simulink model "OpticalFlow"  (Simulink 10.0)
settings: Solver=ode45  StartTime=0.0  StopTime=inf  RelTol=1e-3  EnableMultiTasking=on
undefined symbols (not defined in the file): Horn, Schunck, strel
libraries: vipsnks x4, dspstat3 x2, vipstatistics x1, vipmorphops x1, viptextngfix x1, dspsrcs4 x1, vipanalysis x1
settings Model: Creator=ahwang  LastModifiedBy=bhisma
settings SolverCC: ZeroCrossAlgorithm=Non-adaptive
settings DataIOCC: LimitDataPoints=on  SignalLoggingSaveFormat=ModelDataLogs
settings OptimizationCC: ExpressionDepthLimit=2147483647  InitFltsAndDblsToZero=on
settings DebuggingCC: SolverPrmCheckMsg=warning  FcnCallInpInsideContextMsg=warning  StateNameClashWarn=warning
settings SFSimCC: SimUseLocalCustomCode=on  SimParseCustomCode=off  CustomCodeUndefinedFunction=FilterOut
settings RTWCC: RTWUseLocalCustomCode=on

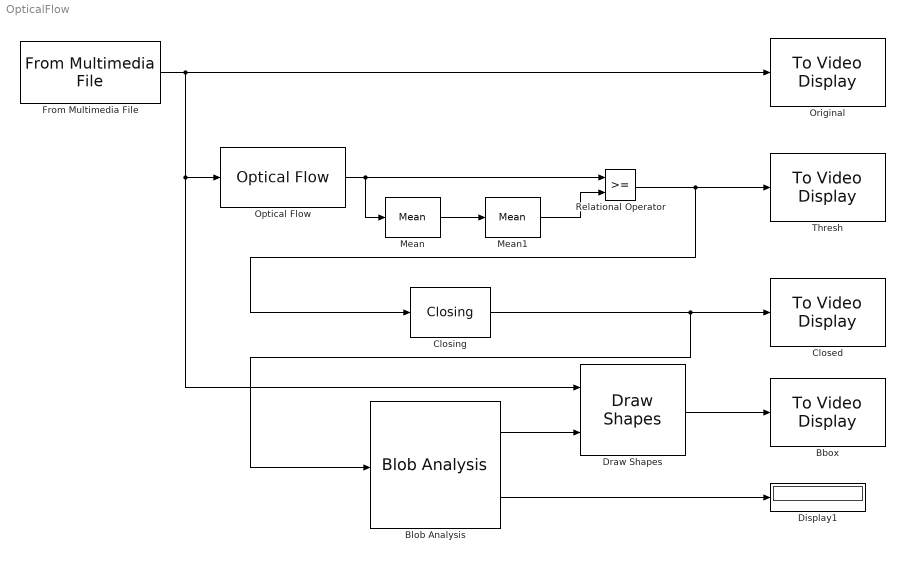
== system OpticalFlow ==
  Bbox : vipsnks/To Video Display  inputType=Obsolete  imagePorts=One multidimensional signal  OutputDevice=On-screen video monitor  fullScreen=off  videoWindowX=289  videoWindowY=479  saveWindowSize=off  videoWindowWidth=44  videoWindowHeight=41  dataOrg=Column-major
      settings: SourceProductName=Computer Vision Toolbox  SourceProductBaseCode=VP
  Blob Analysis : vipstatistics/Blob Analysis  area=off  centroid=off  bBox=on  majorAxis=off  minorAxis=off  angle=off  eccentricity=off  equivDiameterSq=off  extent=off  perimeter=off  maxBlobs=50  warnIfNumBlobsExceeded=on  isCount=on  useMinArea=on  minArea=200  useMaxArea=off  maxArea=intmax('uint32')  excludeBorderBlob=off  outDT=double  isOutVarDim=off  isFill=on  fillValues=-1  conn=8  isLabel=off  outputMode=Binary point scaling  outputWordLength=32  outputFracLength=16  firstCoeffMode=Binary point scaling  firstCoeffWordLength=16  firstCoeffFracLength=14  secondCoeffMode=Binary point scaling  secondCoeffWordLength=32  secondCoeffFracLength=16  accumMode=Binary point scaling  accumWordLength=32  accumFracLength=0  prodOutputMode=Binary point scaling  prodOutputWordLength=32  prodOutputFracLength=16  roundingMode=Floor  overflowMode=off
      settings: SourceProductName=Computer Vision Toolbox  SourceProductBaseCode=VP
  Closed : vipsnks/To Video Display  inputType=Obsolete  imagePorts=One multidimensional signal  OutputDevice=On-screen video monitor  fullScreen=off  videoWindowX=292  videoWindowY=332  saveWindowSize=off  videoWindowWidth=44  videoWindowHeight=41  dataOrg=Column-major
      settings: SourceProductName=Computer Vision Toolbox  SourceProductBaseCode=VP
  Closing : vipmorphops/Closing  nhoodsrc=Specify via dialog  strel=strel('disk',5)
      settings: SourceProductName=Computer Vision Toolbox  SourceProductBaseCode=VP
  Display1 : Display
  Draw Shapes : viptextngfix/Draw Shapes  shape=Rectangles  fill=off  display=Black  intensity=200  color=[200 255 100]  opacity=0.6  viewport=Entire image  antialiasing=off  inType=Obsolete  imagePorts=One multidimensional signal
      settings: SourceProductName=Computer Vision Toolbox  SourceProductBaseCode=VP
  From Multimedia File : dspsrcs4/From Multimedia File  inputFilename=viptraffic.avi  loop=on  numPlays=inf  outputStreams=Video only  videoDataType=double  audioDataType=int16  inheritSampleTime=on  userDefinedSampleTime=1/30  noAudioOutput=off  isIntensityVideo=on  colorVideoFormat=One multidimensional signal  outputEOF=off  dataOrg=Column-major
      settings: SourceProductName=DSP System Toolbox  SourceProductBaseCode=DS
  Mean : dspstat3/Mean  run=off  reset_popup=None  directionMode=Entire input  dimension=1  treatSBRowAsCol=on  roiEnable=off  roiType=Rectangles  roiPortion=Entire ROI  roiOutput=Individual statistics for each ROI  roiFlag=off  roundingMode=Floor  overflowMode=off
  Mean1 : dspstat3/Mean  run=on  reset_popup=None  directionMode=Entire input  dimension=1  treatSBRowAsCol=on  roiEnable=off  roiType=Rectangles  roiPortion=Entire ROI  roiOutput=Individual statistics for each ROI  roiFlag=off  roundingMode=Floor  overflowMode=off
  Optical Flow : vipanalysis/Optical Flow  SystemSampleTime=-1  method=Horn-Schunck  gradMethod=Difference filter [-1 1]  which2img=Current frame and N-th frame back  N=1  outVelForm=Magnitude-squared  lambda=1  stop_criteria=When maximum number of iterations is reached  maxAllowAbsDiff=eps  maxIter=10  numInports=3  sigmaS=1.5  sigmaW=1  eigTh=0.0039  discardNormalFlow=off  outputCurrentImage=off  prodOutputMode=Binary point scaling  prodOutputWordLength=32  prodOutputFracLength=20  outputMode=Binary point scaling  outputWordLength=32  outputFracLength=20  roundingMode=Nearest  overflowMode=on
      settings: SourceProductName=Computer Vision Toolbox  SourceProductBaseCode=VP
  Original : vipsnks/To Video Display  inputType=Obsolete  imagePorts=One multidimensional signal  OutputDevice=On-screen video monitor  fullScreen=off  videoWindowX=292  videoWindowY=32  saveWindowSize=off  videoWindowWidth=44  videoWindowHeight=41  dataOrg=Column-major
      settings: SourceProductName=Computer Vision Toolbox  SourceProductBaseCode=VP
  Relational Operator : RelationalOperator  OutDataTypeStr=boolean  RndMeth=Nearest
  Thresh : vipsnks/To Video Display  inputType=Obsolete  imagePorts=One multidimensional signal  OutputDevice=On-screen video monitor  fullScreen=off  videoWindowX=292  videoWindowY=180  saveWindowSize=off  videoWindowWidth=44  videoWindowHeight=41  dataOrg=Column-major
      settings: SourceProductName=Computer Vision Toolbox  SourceProductBaseCode=VP
  wires:
  From Multimedia File/1 -> Original/1, Optical Flow/1, Draw Shapes/1
  Optical Flow/1 -> Relational Operator/1, Mean/1
  Mean/1 -> Mean1/1
  Relational Operator/1 -> Thresh/1, Closing/1
  Mean1/1 -> Relational Operator/2
  Closing/1 -> Closed/1, Blob Analysis/1
  Blob Analysis/1 -> Draw Shapes/2
  Blob Analysis/2 -> Display1/1
  Draw Shapes/1 -> Bbox/1
